simulink model "sensorless_by_estimated_rotate"  (R2025a)
settings: Solver=ode4  StartTime=0.0  StopTime=1  FixedStep=step_time  MaxStep=1e-4  MinStep=1e-6
values from neighbouring files (symbols this model uses):
  B = 0.0001    [Copy_of_main.m]    (also in main.m)
  init_Thetar = 20 *(pi/180)    (= 0.349065850399)    [Copy_of_main.m]    (also in main.m)
  Is_rated = 10    [Copy_of_main.m]    (also in main.m)
  J = 0.045    [Copy_of_main.m]    (also in main.m)
  K = 2.6    [Copy_of_main.m]    (also in main.m)
  Kas = 1/Kps    (= 1.01859163579)    [Copy_of_main.m]    (also in main.m)
  Kic = Rs*Wcc    (= 1256.63706144)    [Copy_of_main.m]    (also in main.m)
  Kis = J*Wsc^2/5/Kt    (= 6.16850275068)    [Copy_of_main.m]    (also in main.m)
  Kpc = Lds*Wcc    (= 18.8495559215)    [Copy_of_main.m]    (also in main.m)
  Kps = J*Wsc/Kt    (= 0.981747704247)    [Copy_of_main.m]    (also in main.m)
  Lamf = 0.12    [Copy_of_main.m]    (also in main.m)
  Lds = 30.0e-3    (= 0.03)    [Copy_of_main.m]    (also in main.m)
  Lqs = 40.0e-3    (= 0.04)    [Copy_of_main.m]    (also in main.m)
  mm = 2    [Copy_of_main.m]    (also in main.m)
  Mode = 2    [Copy_of_main.m]    (also in main.m)
  P = 8    [Copy_of_main.m]    (also in main.m)
  Rs = 2    [Copy_of_main.m]    (also in main.m)
  Thetar_hat_init = 0    [Copy_of_main.m]    (also in main.m)
  V_inj = 35    [Copy_of_main.m]    (also in main.m)
  w_h = 2*pi*5000    (= 31415.9265359)    [Copy_of_main.m]    (also in main.m)
  zeta = 0.8    [Copy_of_main.m]    (also in main.m)
settings Model: Creator=moon  LastModifiedBy=New
settings RTWCC: GPUComputeCapability=3.5

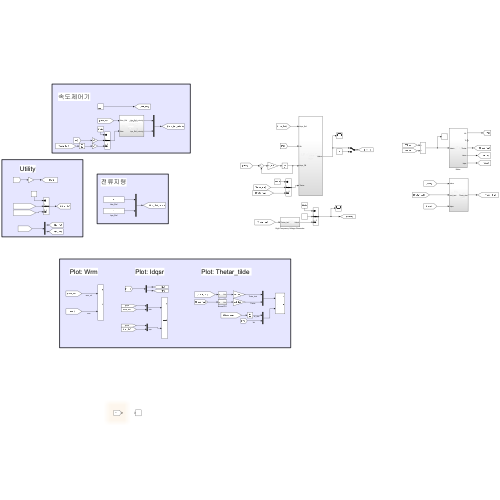
[thumbnail: Simulink's stored preview of the top-level diagram]
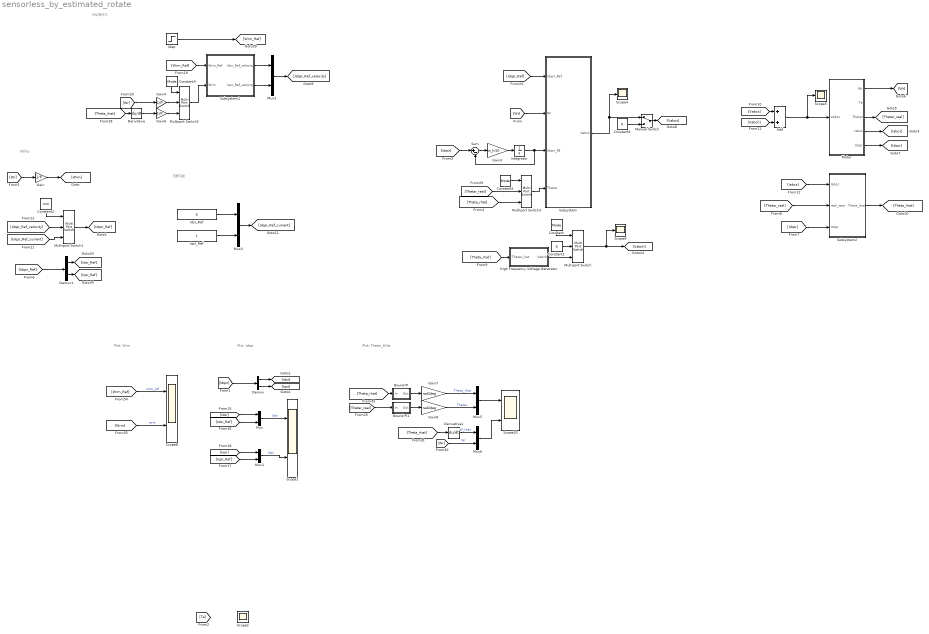
== system sensorless_by_estimated_rotate ==
  note: Plot: Thetar_tilde
  note: 전류지령
  note: 속도제어기
  note: Plot: Wrm
  note: Plot: Idqsr
  note: Utility
  Add : Sum
  Bound PI : Subsystem
  Bound PI1 : Subsystem
  Constant : Constant  Value=Mode
  Constant1 : Constant  Value=0
  Constant2 : Constant  Value=mm
  Constant3 : Constant  Value=0
  Constant4 : Constant  Value=Mode
  Constant5 : Constant  Value=Mode
  Demux : Demux  Outputs=2
  Demux1 : Demux  Outputs=2
  Derivative : Derivative
  Derivative1 : Derivative
  Gain : Gain  Gain=1/P
  Gain3 : Gain  Gain=w_h/10
  Gain4 : Gain  Gain=1/P
  Gain6 : Gain  Gain=1/P
  Gain7 : Gain  Gain=rad2deg
  Gain8 : Gain  Gain=rad2deg
  High Frequency Voltage Generator : Subsystem
  Idsr_Ref : Constant  Value=0
  Integrator : Integrator
  Iqsr_Ref : Constant
  Manual Switch : ManualSwitch
  Motor : Subsystem
  Multiport Switch{,1..3} (4 alike) : MultiPortSwitch  Inputs=2  SaturateOnIntegerOverflow=off  InputSameDT=off
  Mux{,1..3,5..6} (6 alike) : Mux  Inputs=2
  Scope1 : Scope  NumInputPorts=2
      settings: ActiveDisplayYMinimum=-0.50504095999348508  ActiveDisplayYMaximum=4.5453686399413664  DataLoggingVariableName=ScopeData8
  Scope10 : Scope  NumInputPorts=2
      settings: ActiveDisplayYMinimum=-224.98670560770961  ActiveDisplayYMaximum=224.99571861056438  DataLoggingVariableName=ScopeData18
  Scope{2,4..5,9} (4 alike) : Scope
      Scope2 settings: DataLoggingVariableName=ScopeData10
      Scope4 settings: ActiveDisplayYMinimum=-31.981460446682071  ActiveDisplayYMaximum=40.325933755700383  DataLoggingVariableName=ScopeData12
      Scope5 settings: ActiveDisplayYMinimum=-27773.707883194304  ActiveDisplayYMaximum=27837.048942694244  DataLoggingVariableName=ScopeData14
      Scope9 settings: ActiveDisplayYMinimum=-37.647694809538308  ActiveDisplayYMaximum=38.549948693412333  DataLoggingVariableName=ScopeData17
  Scope8 : Scope  NumInputPorts=2
      settings: ActiveDisplayYMinimum=-8.7705192638891525  ActiveDisplayYMaximum=71.436735374708334
  Step : Step  Time=0.1  After=5  SampleTime=0
  Subsystem : Subsystem
  Subsystem1 : Subsystem
  Subsystem2 : Subsystem
  Sum : Sum  Inputs=|+-
  wires:
  [Wrm_Ref] -> Scope8/1  "wrm_ref"
  [Wrm] -> Scope8/2  "wrm"
  Step/1 -> [Wrm_Ref]
  Motor/3(Thetar) -> [Thetar_real]
  Motor/1(Wr) -> [Wr]
  Add/1 -> Motor/1(Vabcs), Scope5/1
  Motor/5(Idqsr) -> [Idqsr]
  [Wr] -> Subsystem/2(Wr)
  Subsystem/1(Vabcs) -> Scope4/1, Manual Switch/1
  [Wr] -> Gain/1
  Gain/1 -> [Wrm]
  Subsystem2/1(Theta_rhat) -> [Theta_rhat]
  High Frequency Voltage Generator/1(Vabch) -> Multiport Switch/3
  Constant1/1 -> Multiport Switch/2
  Constant/1 -> Multiport Switch/1
  [Vabch] -> Add/2
  [Vabcs] -> Add/1
  Multiport Switch/1 -> Scope9/1, [Vabch]
  [Idqsr] -> Demux/1
  Demux/1 -> [Idsr]
  Demux/2 -> [Iqsr]
  [Idsr] -> Mux/1
  Mux/1 -> Scope1/1  "Idsr"
  Mux1/1 -> Scope1/2  "Iqsr"
  [Idsr_Ref] -> Mux/2
  [Iqsr] -> Mux1/1
  [Wrm_Ref] -> Subsystem1/1(Wrm_Ref)
  Subsystem1/1(Idsr_Ref_velocity) -> Mux2/1
  Subsystem1/2(Iqsr_Ref_velocity) -> Mux2/2
  Mux2/1 -> [Idqsr_Ref_velocity]
  Iqsr_Ref/1 -> Mux3/2
  Idsr_Ref/1 -> Mux3/1
  Mux3/1 -> [Idqsr_Ref_current]
  Constant2/1 -> Multiport Switch1/1
  [Idqsr_Ref_velocity] -> Multiport Switch1/2
  [Idqsr_Ref_current] -> Multiport Switch1/3
  Multiport Switch1/1 -> [Idqsr_Ref]
  [Iqsr_Ref] -> Mux1/2
  [Theta_rhat] -> High Frequency Voltage Generator/1(Thetar_hat)
  [Thetar_real] -> Subsystem2/2(real_test)
  Manual Switch/1 -> [Vabcs]
  Constant3/1 -> Manual Switch/2
  Gain3/1 -> Integrator/1
  Sum/1 -> Gain3/1
  [Idqsr_Ref] -> Subsystem/1(Idqsr_Ref)
  Multiport Switch2/1 -> Subsystem1/2(Wrm)
  [Wr] -> Gain4/1
  Constant4/1 -> Multiport Switch2/1
  [Theta_rhat] -> Derivative/1
  Derivative/1 -> Gain6/1
  Constant5/1 -> Multiport Switch3/1
  [Thetar_real] -> Multiport Switch3/2
  [Theta_rhat] -> Multiport Switch3/3
  Multiport Switch3/1 -> Subsystem/4(Thetar)
  [Idqsr] -> Sum/1
  Integrator/1 -> Sum/2, Subsystem/3(Idqsr_FB)
  Gain4/1 -> Multiport Switch2/2
  Gain6/1 -> Multiport Switch2/3
  Bound PI/1(Out) -> Gain7/1
  Mux5/1 -> Scope10/1
  [Thetar_real] -> Bound PI1/1(In)
  [Theta_rhat] -> Bound PI/1(In)
  Gain7/1 -> Mux5/1  "Theta_rhat"
  Gain8/1 -> Mux5/2  "Thetar"
  Bound PI1/1(Out) -> Gain8/1
  [Wr] -> Mux6/2  "Wr"
  [Theta_rhat] -> Derivative1/1
  Derivative1/1 -> Mux6/1  "W_rhat"
  Mux6/1 -> Scope10/2
  Demux1/2 -> [Iqsr_Ref]
  Demux1/1 -> [Idsr_Ref]
  [Idqsr_Ref] -> Demux1/1
  Motor/4(Iabcs) -> [Iabcs]
  [Iabcs] -> Subsystem2/1(Iabcs)
  [Idqsr] -> Subsystem2/3(Idqsr)

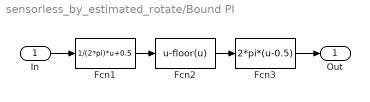
== system sensorless_by_estimated_rotate/Bound PI ==
  In : Inport
  Fcn1 : Fcn  Expr=1/(2*pi)*u+0.5
  Fcn2 : Fcn  Expr=u-floor(u)
  Fcn3 : Fcn  Expr=2*pi*(u-0.5)
  Out : Outport
  wires:
  Fcn1/1 -> Fcn2/1
  Fcn2/1 -> Fcn3/1
  In/1 -> Fcn1/1
  Fcn3/1 -> Out/1

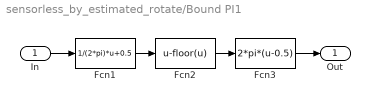
== system sensorless_by_estimated_rotate/Bound PI1 ==
  In : Inport
  Fcn1 : Fcn  Expr=1/(2*pi)*u+0.5
  Fcn2 : Fcn  Expr=u-floor(u)
  Fcn3 : Fcn  Expr=2*pi*(u-0.5)
  Out : Outport
  wires:
  Fcn3/1 -> Out/1
  In/1 -> Fcn1/1
  Fcn2/1 -> Fcn3/1
  Fcn1/1 -> Fcn2/1

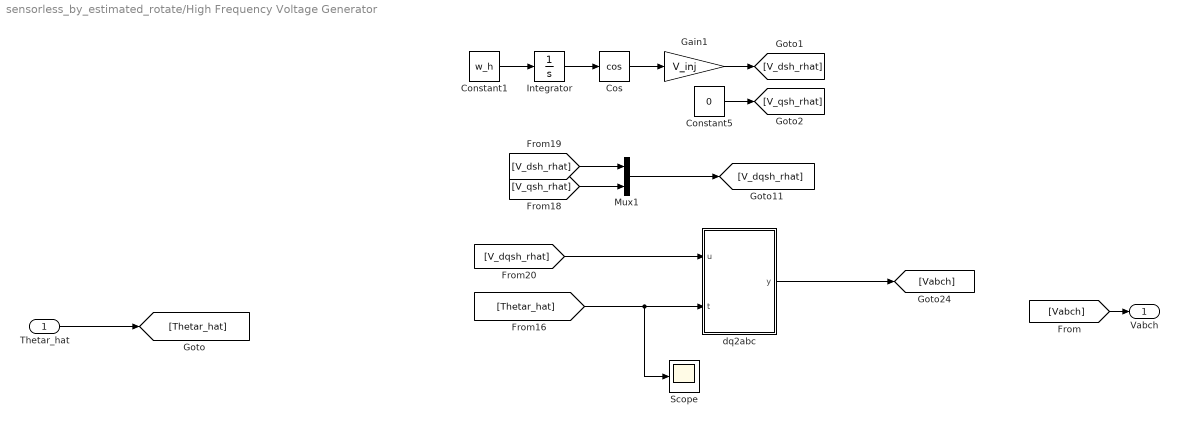
== system sensorless_by_estimated_rotate/High Frequency Voltage Generator ==
  Thetar_hat : Inport
  Constant1 : Constant  Value=w_h
  Constant5 : Constant  Value=0
  Cos : Trigonometry  Operator=cos
  Gain1 : Gain  Gain=V_inj
  Integrator : Integrator
  Mux1 : Mux  Inputs=2
  Scope : Scope
      settings: ActiveDisplayYMinimum=-1  ActiveDisplayYMaximum=1  DataLoggingVariableName=ScopeData6
  dq2abc : MATLAB Function  TreatAsAtomicUnit=on
  Vabch : Outport
  wires:
  Constant5/1 -> [V_qsh_rhat]
  Integrator/1 -> Cos/1
  Constant1/1 -> Integrator/1
  Mux1/1 -> [V_dqsh_rhat]
  Gain1/1 -> [V_dsh_rhat]
  dq2abc/1(y) -> [Vabch]
  [Thetar_hat] -> Scope/1, dq2abc/2(t)
  Cos/1 -> Gain1/1
  [V_dsh_rhat] -> Mux1/1
  [V_qsh_rhat] -> Mux1/2
  [V_dqsh_rhat] -> dq2abc/1(u)
  [Vabch] -> Vabch/1
  Thetar_hat/1 -> [Thetar_hat]

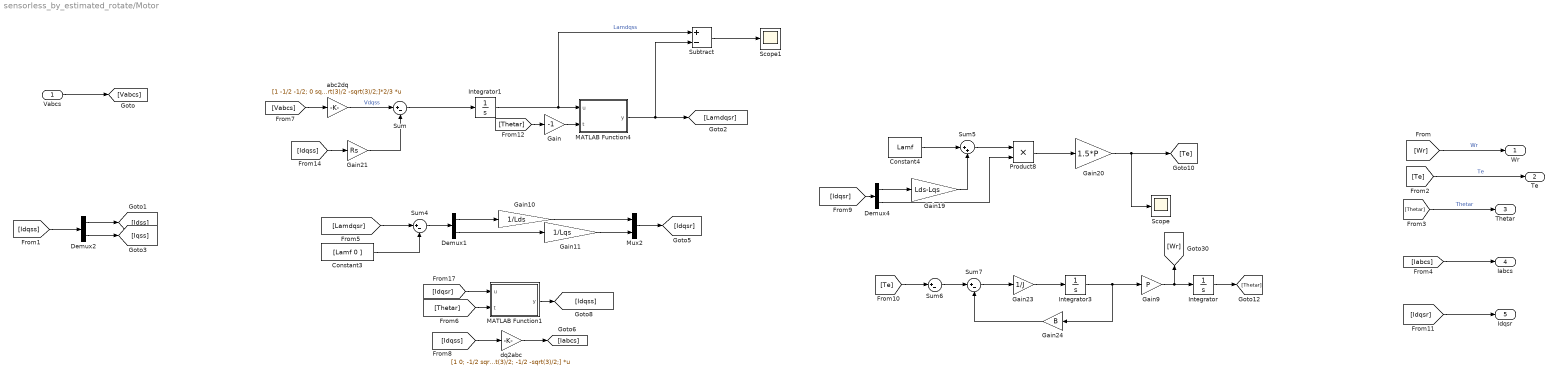
== system sensorless_by_estimated_rotate/Motor ==
  Vabcs : Inport
  Constant3 : Constant  Value=[Lamf 0 ]
  Constant4 : Constant  Value=Lamf
  Demux1 : Demux  Outputs=2
  Demux2 : Demux  Outputs=2
  Demux4 : Demux  Outputs=2
  Gain : Gain  Gain=-1
  Gain10 : Gain  Gain=1/Lds
  Gain11 : Gain  Gain=1/Lqs
  Gain19 : Gain  Gain=Lds-Lqs
  Gain20 : Gain  Gain=1.5*P
  Gain21 : Gain  Gain=Rs
  Gain23 : Gain  Gain=1/J
  Gain24 : Gain  Gain=B
  Gain9 : Gain  Gain=P
  Integrator : Integrator  InitialCondition=init_Thetar
  Integrator1 : Integrator
  Integrator3 : Integrator
  MATLAB Function1 : MATLAB Function  TreatAsAtomicUnit=on
  MATLAB Function4 : MATLAB Function  TreatAsAtomicUnit=on
  Mux2 : Mux  Inputs=2
  Product8 : Product
  Scope : Scope
      settings: ActiveDisplayYMinimum=-1  ActiveDisplayYMaximum=1  DataLoggingVariableName=ScopeData2
  Scope1 : Scope
      settings: ActiveDisplayYMinimum=-0.0008172093496326882  ActiveDisplayYMaximum=0.00023756018156422692  DataLoggingVariableName=ScopeData3
  Subtract : Sum  Inputs=+-
  Sum{,4,6..7} (4 alike) : Sum  Inputs=|+-
  Sum5 : Sum  Inputs=|++
  abc2dq : Gain  Gain=[1 -1/2 -1/2; 0 sqrt(3)/2 -sqrt(3)/2;]*2/3  Multiplication=Matrix(K*u)
  dq2abc : Gain  Gain=[1 0; -1/2 sqrt(3)/2; -1/2 -sqrt(3)/2;]  Multiplication=Matrix(K*u)
  Wr : Outport
  Te : Outport  Port=2
  Thetar : Outport  Port=3
  Iabcs : Outport  Port=4
  Idqsr : Outport  Port=5
  wires:
  [Idqsr] -> Demux4/1
  Product8/1 -> Gain20/1
  Sum7/1 -> Gain23/1
  Sum5/1 -> Product8/1
  [Lamdqsr] -> Sum4/1
  [Idqss] -> Gain21/1
  Gain24/1 -> Sum7/2
  Constant4/1 -> Sum5/1
  Demux1/2 -> Gain11/1
  Integrator1/1 -> Subtract/1, MATLAB Function4/1(u)  "Lamdqss"
  Gain23/1 -> Integrator3/1
  Demux1/1 -> Gain10/1
  Gain19/1 -> Sum5/2
  Gain11/1 -> Mux2/2
  Demux4/2 -> Product8/2
  Mux2/1 -> [Idqsr]
  Constant3/1 -> Sum4/2
  Gain10/1 -> Mux2/1
  [Te] -> Sum6/1
  Integrator3/1 -> Gain24/1, Gain9/1
  Sum6/1 -> Sum7/1
  Sum4/1 -> Demux1/1
  Demux4/1 -> Gain19/1
  Vabcs/1 -> [Vabcs]
  [Wr] -> Wr/1  "Wr"
  [Te] -> Te/1  "Te"
  [Thetar] -> Thetar/1  "Thetar"
  [Iabcs] -> Iabcs/1
  [Idqsr] -> Idqsr/1
  abc2dq/1 -> Sum/1  "Vdqss"
  Gain21/1 -> Sum/2
  Integrator/1 -> [Thetar]
  Gain20/1 -> Scope/1, [Te]
  Gain9/1 -> Integrator/1, [Wr]
  [Thetar] -> MATLAB Function1/2(t)
  [Idqsr] -> MATLAB Function1/1(u)
  MATLAB Function1/1(y) -> [Idqss]
  [Idqss] -> dq2abc/1
  dq2abc/1 -> [Iabcs]
  [Vabcs] -> abc2dq/1
  Gain/1 -> MATLAB Function4/2(t)
  [Thetar] -> Gain/1
  MATLAB Function4/1(y) -> Subtract/2, [Lamdqsr]
  Sum/1 -> Integrator1/1
  [Idqss] -> Demux2/1
  Demux2/1 -> [Idss]
  Demux2/2 -> [Iqss]
  Subtract/1 -> Scope1/1

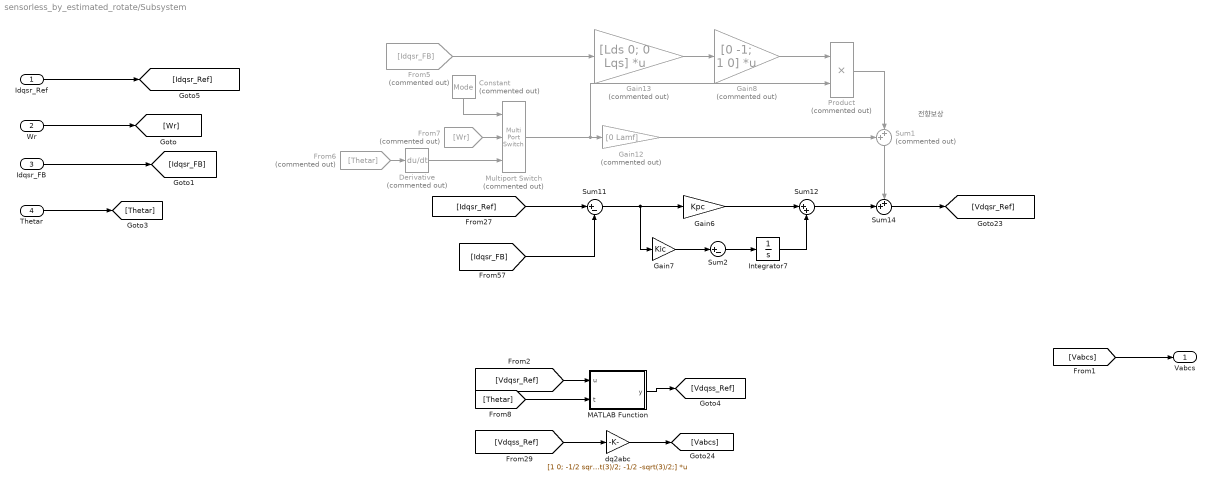
== system sensorless_by_estimated_rotate/Subsystem ==
  note: 전향보상
  Idqsr_Ref : Inport
  Wr : Inport  Port=2
  Idqsr_FB : Inport  Port=3
  Thetar : Inport  Port=4
  Constant : Constant  Commented=on  Value=Mode
  Derivative : Derivative  Commented=on
  From5 : From  Commented=on  GotoTag=Idqsr_FB
  From6 : From  Commented=on  GotoTag=Thetar
  From7 : From  Commented=on  GotoTag=Wr
  Gain12 : Gain  Commented=on  Gain=[0 Lamf]
  Gain13 : Gain  Commented=on  Gain=[Lds 0; 0 Lqs]  Multiplication=Matrix(K*u)
  Gain6 : Gain  Gain=Kpc
  Gain7 : Gain  Gain=Kic
  Gain8 : Gain  Commented=on  Gain=[0 -1; 1 0]  Multiplication=Matrix(K*u)
  Integrator7 : Integrator
  MATLAB Function : MATLAB Function  TreatAsAtomicUnit=on
  Multiport Switch : MultiPortSwitch  Commented=on  Inputs=2  SaturateOnIntegerOverflow=off  InputSameDT=off
  Product : Product  Commented=on
  Sum1 : Sum  Commented=on  Inputs=++|
  Sum11 : Sum  Inputs=|+-
  Sum12 : Sum  Inputs=|++
  Sum14 : Sum  Inputs=++|
  Sum2 : Sum  Inputs=|+-
  dq2abc : Gain  Gain=[1 0; -1/2 sqrt(3)/2; -1/2 -sqrt(3)/2;]  Multiplication=Matrix(K*u)
  Vabcs : Outport
  wires:
  From5/1 -> Gain13/1
  Gain13/1 -> Gain8/1
  Sum12/1 -> Sum14/2
  [Idqsr_FB] -> Sum11/2
  Integrator7/1 -> Sum12/2
  Gain8/1 -> Product/1
  Gain6/1 -> Sum12/1
  Multiport Switch/1 -> Product/2, Gain12/1
  [Idqsr_Ref] -> Sum11/1
  Sum11/1 -> Gain6/1, Gain7/1
  Wr/1 -> [Wr]
  [Vabcs] -> Vabcs/1
  Thetar/1 -> [Thetar]
  Gain7/1 -> Sum2/1
  Sum2/1 -> Integrator7/1
  [Vdqss_Ref] -> dq2abc/1
  dq2abc/1 -> [Vabcs]
  Sum14/1 -> [Vdqsr_Ref]
  Derivative/1 -> Multiport Switch/3
  Constant/1 -> Multiport Switch/1
  From6/1 -> Derivative/1
  From7/1 -> Multiport Switch/2
  Idqsr_Ref/1 -> [Idqsr_Ref]
  Idqsr_FB/1 -> [Idqsr_FB]
  [Vdqsr_Ref] -> MATLAB Function/1(u)
  [Thetar] -> MATLAB Function/2(t)
  MATLAB Function/1(y) -> [Vdqss_Ref]
  Product/1 -> Sum1/2
  Gain12/1 -> Sum1/1
  Sum1/1 -> Sum14/1

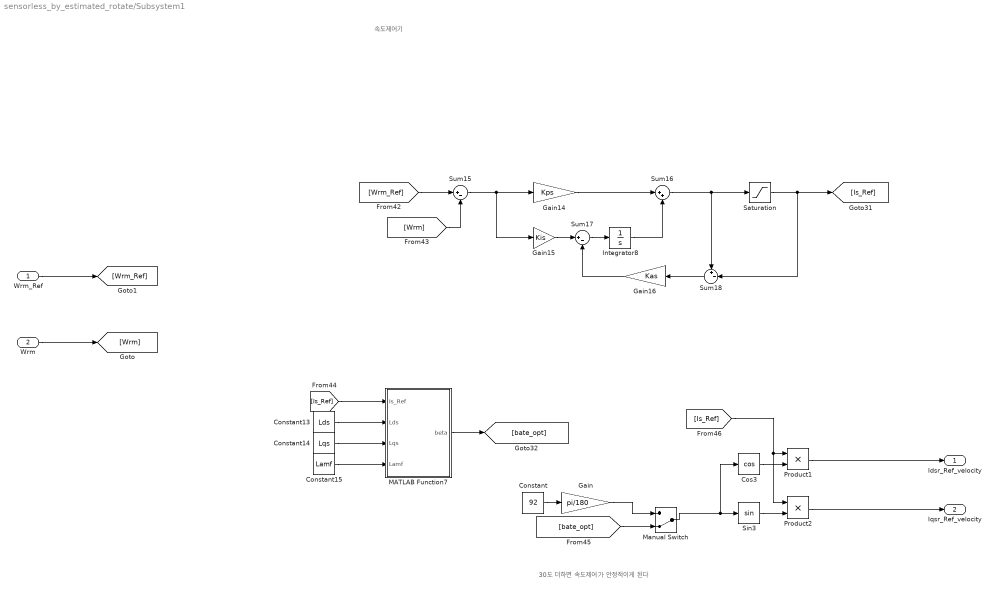
== system sensorless_by_estimated_rotate/Subsystem1 ==
  note: 30도 더하면 속도제어가 안정적이게 된다
  note: 속도제어기
  Wrm_Ref : Inport
  Wrm : Inport  Port=2
  Constant : Constant  Value=92
  Constant13 : Constant  Value=Lds
  Constant14 : Constant  Value=Lqs
  Constant15 : Constant  Value=Lamf
  Cos3 : Trigonometry  Operator=cos
  Gain : Gain  Gain=pi/180
  Gain14 : Gain  Gain=Kps
  Gain15 : Gain  Gain=Kis
  Gain16 : Gain  Gain=Kas
  Integrator8 : Integrator
  MATLAB Function7 : MATLAB Function  TreatAsAtomicUnit=on
  Manual Switch : ManualSwitch  CurrentSetting=0
  Product1 : Product
  Product2 : Product
  Saturation : Saturate  UpperLimit=Is_rated  LowerLimit=-Is_rated
  Sin3 : Trigonometry
  Sum15 : Sum  Inputs=|+-
  Sum16 : Sum  Inputs=|++
  Sum17 : Sum  Inputs=|+-
  Sum18 : Sum  Inputs=+-|
  Idsr_Ref_velocity : Outport
  Iqsr_Ref_velocity : Outport  Port=2
  wires:
  Gain15/1 -> Sum17/1
  [Wrm_Ref] -> Sum15/1
  Saturation/1 -> [Is_Ref], Sum18/2
  Gain16/1 -> Sum17/2
  Sum16/1 -> Saturation/1, Sum18/1
  Product2/1 -> Iqsr_Ref_velocity/1
  Gain14/1 -> Sum16/1
  Product1/1 -> Idsr_Ref_velocity/1
  [Wrm] -> Sum15/2
  Constant14/1 -> MATLAB Function7/3(Lqs)
  [Is_Ref] -> MATLAB Function7/1(Is_Ref)
  Constant13/1 -> MATLAB Function7/2(Lds)
  MATLAB Function7/1(beta) -> [bate_opt]
  Sum18/1 -> Gain16/1
  Sum15/1 -> Gain15/1, Gain14/1
  [Is_Ref] -> Product2/1, Product1/1
  Cos3/1 -> Product1/2
  Sum17/1 -> Integrator8/1
  Manual Switch/1 -> Sin3/1, Cos3/1
  Sin3/1 -> Product2/2
  Integrator8/1 -> Sum16/2
  Constant15/1 -> MATLAB Function7/4(Lamf)
  Wrm/1 -> [Wrm]
  Wrm_Ref/1 -> [Wrm_Ref]
  Constant/1 -> Gain/1
  Gain/1 -> Manual Switch/1
  [bate_opt] -> Manual Switch/2

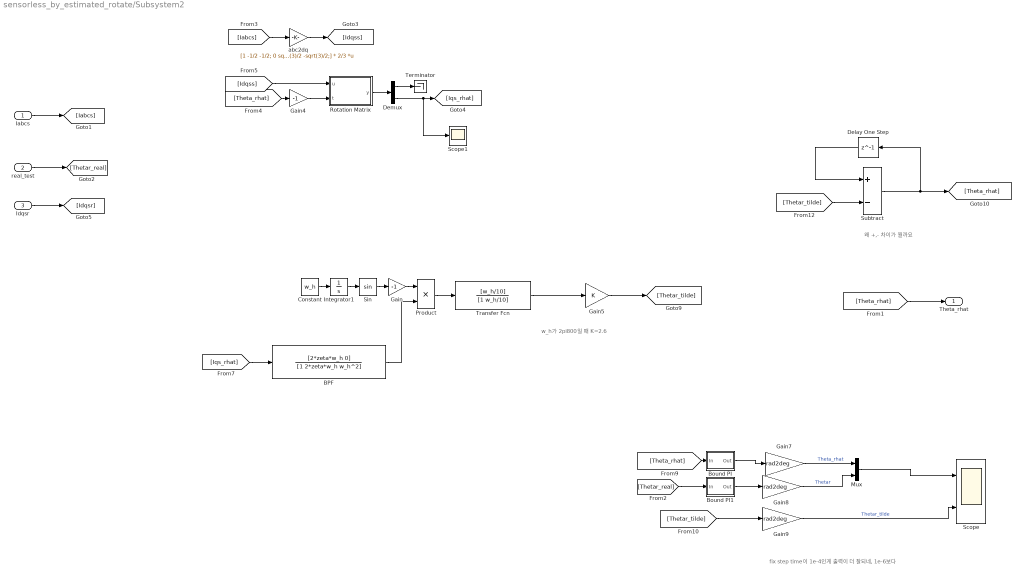
== system sensorless_by_estimated_rotate/Subsystem2 ==
  note: w_h가 2pi800일 때 K=2.6
  note: 왜 +,- 차이가 뭘까요
  note: fix step time이 1e-4인게 출력이 더 잘되네, 1e-6보다
  Iabcs : Inport
  real_test : Inport  Port=2
  Idqsr : Inport  Port=3
  BPF : TransferFcn  Numerator=[2*zeta*w_h 0]  Denominator=[1 2*zeta*w_h w_h^2]
  Bound PI : Subsystem
  Bound PI1 : Subsystem
  Constant : Constant  Value=w_h
  Delay One Step : Delay  DelayLength=1  InitialCondition=Thetar_hat_init
  Demux : Demux  Outputs=2
  Gain : Gain  Gain=-1
  Gain4 : Gain  Gain=-1
  Gain5 : Gain  Gain=K
  Gain7 : Gain  Gain=rad2deg
  Gain8 : Gain  Gain=rad2deg
  Gain9 : Gain  Gain=rad2deg
  Integrator1 : Integrator
  Mux : Mux  Inputs=2
  Product : Product
  Rotation Matrix : MATLAB Function  TreatAsAtomicUnit=on
  Scope : Scope  NumInputPorts=2
      settings: ActiveDisplayYMinimum=-270.07133197247254  ActiveDisplayYMaximum=250.84506508263664  DataLoggingVariableName=ScopeData7
  Scope1 : Scope
      settings: ActiveDisplayYMinimum=-1  ActiveDisplayYMaximum=1
  Sin : Trigonometry
  Subtract : Sum  Inputs=+-
  Terminator : Terminator
  Transfer Fcn : TransferFcn  Numerator=[w_h/10]  Denominator=[1 w_h/10]
  abc2dq : Gain  Gain=[1 -1/2 -1/2; 0 sqrt(3)/2 -sqrt(3)/2;] * 2/3  Multiplication=Matrix(K*u)
  Theta_rhat : Outport
  wires:
  Subtract/1 -> Delay One Step/1, [Theta_rhat]
  Constant/1 -> Integrator1/1
  Demux/2 -> Scope1/1, [Iqs_rhat]
  Rotation Matrix/1(y) -> Demux/1
  Gain4/1 -> Rotation Matrix/2(t)
  Integrator1/1 -> Sin/1
  BPF/1 -> Product/2
  [Thetar_tilde] -> Subtract/2
  Demux/1 -> Terminator/1
  Sin/1 -> Gain/1
  [Theta_rhat] -> Gain4/1
  [Idqss] -> Rotation Matrix/1(u)
  Iabcs/1 -> [Iabcs]
  [Theta_rhat] -> Theta_rhat/1
  Gain/1 -> Product/1
  Delay One Step/1 -> Subtract/1
  real_test/1 -> [Thetar_real]
  [Thetar_real] -> Bound PI1/1(In)
  Mux/1 -> Scope/1
  Product/1 -> Transfer Fcn/1
  [Iqs_rhat] -> BPF/1
  Gain7/1 -> Mux/1  "Theta_rhat"
  Gain8/1 -> Mux/2  "Thetar"
  [Theta_rhat] -> Bound PI/1(In)
  [Thetar_tilde] -> Gain9/1
  Gain9/1 -> Scope/2  "Thetar_tilde"
  Bound PI/1(Out) -> Gain7/1
  Bound PI1/1(Out) -> Gain8/1
  abc2dq/1 -> [Idqss]
  [Iabcs] -> abc2dq/1
  Idqsr/1 -> [Idqsr]
  Transfer Fcn/1 -> Gain5/1
  Gain5/1 -> [Thetar_tilde]

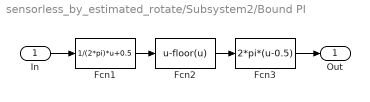
== system sensorless_by_estimated_rotate/Subsystem2/Bound PI ==
  In : Inport
  Fcn1 : Fcn  Expr=1/(2*pi)*u+0.5
  Fcn2 : Fcn  Expr=u-floor(u)
  Fcn3 : Fcn  Expr=2*pi*(u-0.5)
  Out : Outport
  wires:
  Fcn1/1 -> Fcn2/1
  Fcn2/1 -> Fcn3/1
  In/1 -> Fcn1/1
  Fcn3/1 -> Out/1

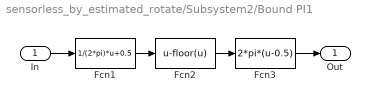
== system sensorless_by_estimated_rotate/Subsystem2/Bound PI1 ==
  In : Inport
  Fcn1 : Fcn  Expr=1/(2*pi)*u+0.5
  Fcn2 : Fcn  Expr=u-floor(u)
  Fcn3 : Fcn  Expr=2*pi*(u-0.5)
  Out : Outport
  wires:
  Fcn3/1 -> Out/1
  In/1 -> Fcn1/1
  Fcn2/1 -> Fcn3/1
  Fcn1/1 -> Fcn2/1

== matlab function sensorless_by_estimated_rotate/Motor/MATLAB Function1 ==
  data: u input; y output; t input
function y = fcn(u,t)

R = [cos(t) -sin(t); sin(t) cos(t)];



y = R * u;

== matlab function sensorless_by_estimated_rotate/Subsystem/MATLAB Function ==
  data: u input; y output; t input
function y = fcn(u,t)

R=[cos(t) -sin(t); sin(t) cos(t)];


y = R*u;

== matlab function sensorless_by_estimated_rotate/Subsystem2/Rotation Matrix ==
  data: u input size=[2 1]; y output size=[2 1]; t input
function y = fcn(u, t)

R = [cos(t) -sin(t); sin(t) cos(t)];

y = R*u;

== matlab function sensorless_by_estimated_rotate/Subsystem1/MATLAB Function7 ==
  data: Is_Ref input; beta output; Lds input; Lqs input; Lamf input
function beta = fcn(Is_Ref, Lds, Lqs, Lamf)

beta = acos((-Lamf+sqrt(Lamf^2+8*(Lds-Lqs)^2*Is_Ref^2))/(4*(Lds-Lqs)*(Is_Ref+eps)));

== matlab function sensorless_by_estimated_rotate/Motor/MATLAB Function4 ==
  data: u input; y output; t input
function y = fcn(u,t)

R = [cos(t) -sin(t); sin(t) cos(t)];



y = R * u;

== matlab function sensorless_by_estimated_rotate/High Frequency Voltage Generator/dq2abc ==
  data: u input size=[2 1]; y output size=[3 1]; t input
function y = fcn(u, t)

a=2*pi/3;

TT = @(t) ...
    [cos(t)  cos(t-a)  cos(t+a);
    -sin(t) -sin(t-a) -sin(t+a);
        1/2       1/2       1/2;] *2/3;

y = TT(t) \ [u; 0];
